simulink model "Task_2"  (R2020a)
settings: Solver=VariableStepAuto  StartTime=0.0  StopTime=1000  RelTol=1e-3
settings Model: Creator=dvdia  LastModifiedBy=dvdia

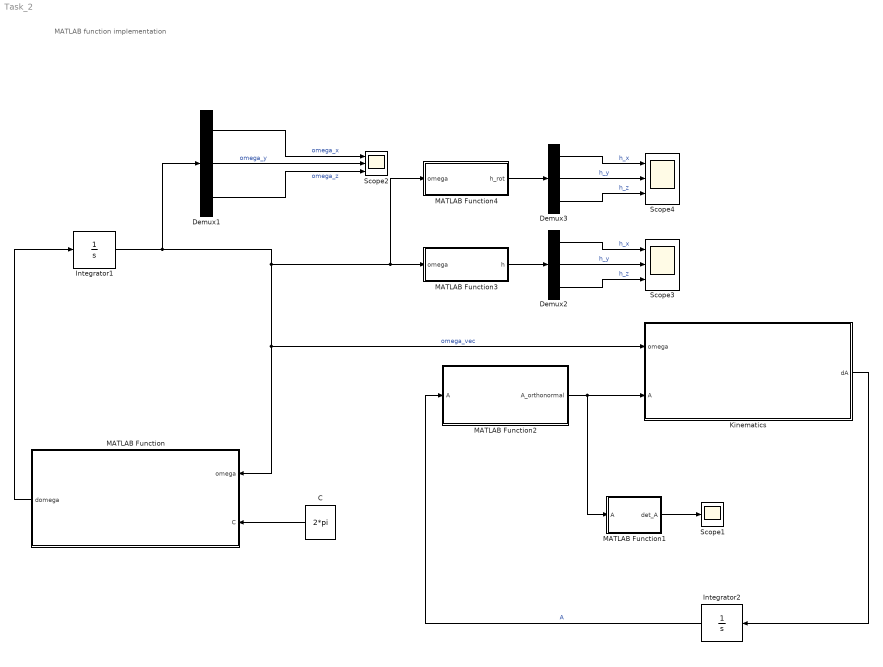
== system Task_2 ==
  note: MATLAB function implementation
  C : Constant  Value=2*pi
  Demux1 : Demux  Outputs=3
  Demux2 : Demux  Outputs=3
  Demux3 : Demux  Outputs=3
  Integrator1 : Integrator  InitialCondition="[ 2*pi  1.e-2 1e-2]"
  Integrator2 : Integrator  InitialCondition=eye(3)
  Kinematics : MATLAB Function  TreatAsAtomicUnit=on
  MATLAB Function : MATLAB Function  TreatAsAtomicUnit=on
  MATLAB Function1 : MATLAB Function  TreatAsAtomicUnit=on
  MATLAB Function2 : MATLAB Function  TreatAsAtomicUnit=on
  MATLAB Function3 : MATLAB Function  TreatAsAtomicUnit=on
  MATLAB Function4 : MATLAB Function  TreatAsAtomicUnit=on
  Scope1 : Scope
  Scope2 : Scope  NumInputPorts=3
  Scope3 : Scope  NumInputPorts=3
  Scope4 : Scope  NumInputPorts=3
  wires:
  Demux1/2 -> Scope2/2  "omega_y"
  MATLAB Function/1(domega) -> Integrator1/1
  Demux1/1 -> Scope2/1  "omega_x"
  Integrator1/1 -> Demux1/1, MATLAB Function4/1(omega), MATLAB Function3/1(omega), MATLAB Function/1(omega), Kinematics/1(omega)  "omega_vec"
  Demux1/3 -> Scope2/3  "omega_z"
  Integrator2/1 -> MATLAB Function2/1(A)  "A"
  Kinematics/1(dA) -> Integrator2/1
  MATLAB Function1/1(det_A) -> Scope1/1
  MATLAB Function2/1(A_orthonormal) -> MATLAB Function1/1(A), Kinematics/2(A)
  MATLAB Function3/1(h) -> Demux2/1
  Demux2/2 -> Scope3/2  "h_y"
  Demux2/1 -> Scope3/1  "h_x"
  Demux2/3 -> Scope3/3  "h_z"
  Demux3/3 -> Scope4/3  "h_z"
  Demux3/1 -> Scope4/1  "h_x"
  Demux3/2 -> Scope4/2  "h_y"
  MATLAB Function4/1(h_rot) -> Demux3/1
  C/1 -> MATLAB Function/2(C)

== matlab function Task_2/MATLAB Function ==
  data: omega input; domega output; C input
function domega = fcn(omega,C)

% Inertia moments

I_x = 0.07;         %  [kg*m^2]
I_y = 0.0504;       %  [kg*m^2]
I_z = 0.0109;       %  [kg*m^2]


% Initial conditions

%C = 2*pi;
% C = 0.1;
% C = 1;
% C = 1.5;
% C = 2;
omega0_vec = [C 1.e-2 1e-2];

% Set omegas
omega_x = omega(1);
omega_y = omega(2);
omega_z = omega(3);


% Compute d_omegas
domega_x = (I_y-I_z)*omega_y*omega_z/I_x;
domega_y = (I_z-I_x)*omega_x*omega_z;
domega_z = (I_x - I_y)*omega_y*omega_x / I_z;
domega = [ domega_x domega_y domega_z ];
end

== matlab function Task_2/MATLAB Function1 ==
  data: A input; det_A output
function det_A = fcn(A)

det_A = det(A);

== matlab function Task_2/MATLAB Function2 ==
  data: A input; A_orthonormal output
function A_orthonormal = orthonormilizer(A)

% Iterative formulas for orthonormalization
% first order approximation: single step iteration
A_orthonormal = A*3/2 - A*(A')*A/2;

end

== matlab function Task_2/MATLAB Function3 ==
  data: omega input; h output
function h = ang_mom(omega)
% Inertia moments

I_x = 0.07;         %  [kg*m^2]
I_y = 0.0504;       %  [kg*m^2]
I_z = 0.0109;       %  [kg*m^2]

I = diag([I_x I_y I_z]);

h = I*omega;

end

== matlab function Task_2/MATLAB Function4 ==
  data: omega input; h_rot output
function h_rot = rot_ang_mom(omega)
% Inertia moments

I_x = 0.07;         %  [kg*m^2]
I_y = 0.0504;       %  [kg*m^2]
I_z = 0.0109;       %  [kg*m^2]

I = diag([I_x I_y I_z]);

h = I*omega;

h_b = 
% rotation about z of pi/2
theta = pi/2;

% rotation matrix for rotating a vector
% around z
B = [   cos(theta)  -sin(theta) 0
        sin(theta)  cos(theta)  0
        0           0           1   ];
    
h_rot = B*h;
end

== matlab function Task_2/Kinematics ==
  data: omega input; dA output; A input
function dA = fcn(omega,A)


omega_x = omega(1);
omega_y = omega(2);
omega_z = omega(3);

w_cross = [ 0 -omega_z omega_y
            omega_z 0 -omega_x
            -omega_y omega_x 0 ];
        
dA = - w_cross * A ;
end
